simulink library "planarWaveModel_ul"  (R2018b)
settings: Solver=VariableStepAuto  StartTime=0.0  StopTime=10.0  RelTol=1e-3
undefined symbols (not defined in the file): env
settings Model: Creator=jcreed2  LastModifiedBy=jcreed2

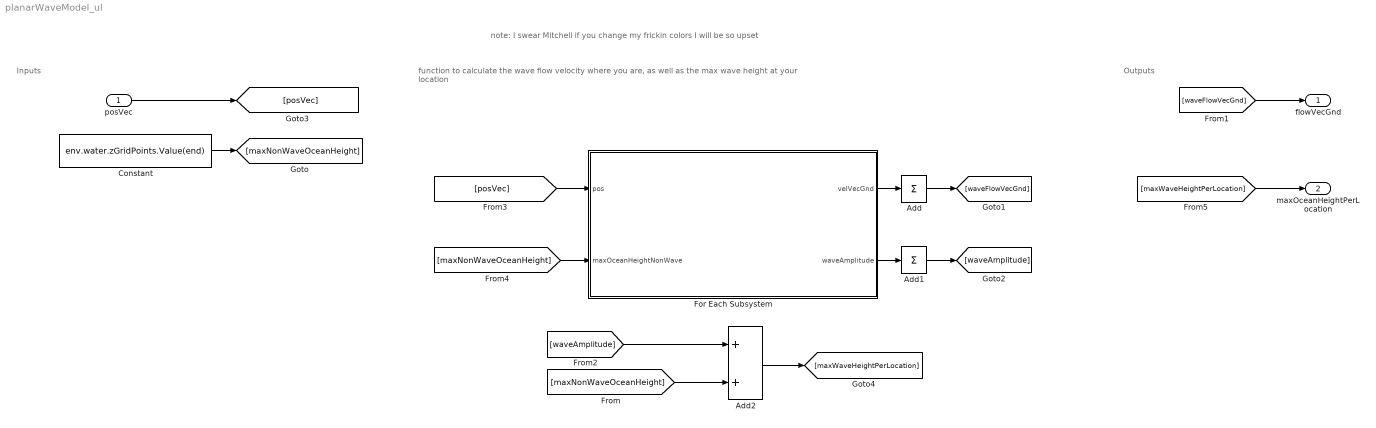
== system planarWaveModel_ul ==
  note: note: I swear Mitchell if you change my frickin colors I will be so upset
  note: Outputs
  note: Inputs
  note: function to calculate the wave flow velocity where you are, as well as the max wave height at your location
  posVec : Inport
  Add : Sum  Inputs=+
  Add1 : Sum  Inputs=+
  Add2 : Sum
  Constant : Constant  Value=env.water.zGridPoints.Value(end)
  For Each Subsystem : Subsystem  TreatAsAtomicUnit=on  mask{waveStruct=env.waterWave.struct('ENV.planarWaveModel')}
      mask prompts: waveStruct "wave structure"
      mask DialogControl Control2 Prompt: Insert wave structure
  "flowVecGnd " : Outport
  maxOceanHeightPerLocation : Outport  Port=2
  wires:
  Constant/1 -> [maxNonWaveOceanHeight]
  For Each Subsystem/1("velVecGnd ") -> Add/1
  For Each Subsystem/2(waveAmplitude) -> Add1/1
  Add/1 -> [waveFlowVecGnd]
  [waveFlowVecGnd] -> "flowVecGnd "/1
  Add1/1 -> [waveAmplitude]
  posVec/1 -> [posVec]
  [posVec] -> For Each Subsystem/1("pos ")
  [waveAmplitude] -> Add2/1
  [maxNonWaveOceanHeight] -> Add2/2
  [maxNonWaveOceanHeight] -> For Each Subsystem/2("maxOceanHeightNonWave ")
  Add2/1 -> [maxWaveHeightPerLocation]
  [maxWaveHeightPerLocation] -> maxOceanHeightPerLocation/1

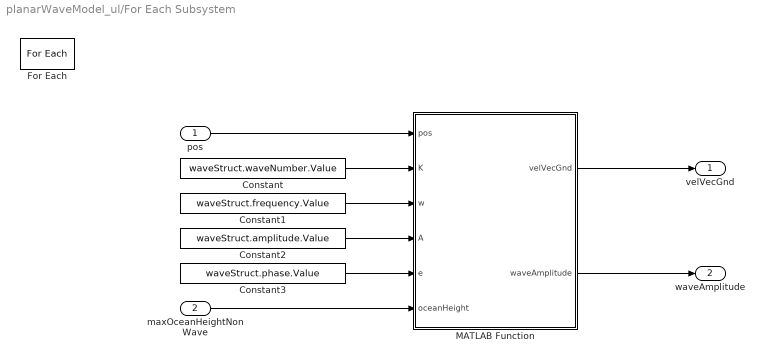
== system planarWaveModel_ul/For Each Subsystem ==
  "pos " : Inport
  "maxOceanHeightNonWave " : Inport  Port=2
  Constant : Constant  Value=waveStruct.waveNumber.Value
  Constant1 : Constant  Value=waveStruct.frequency.Value
  Constant2 : Constant  Value=waveStruct.amplitude.Value
  Constant3 : Constant  Value=waveStruct.phase.Value
  For Each : ForEach  DisableCoverage=on  IterateSubsysMaskParameter=on  SubsysMaskParameterIterationDimension=2  IndexMode=One-based
  MATLAB Function : MATLAB Function  TreatAsAtomicUnit=on
  "velVecGnd " : Outport  ConcatenationDimension=1
  waveAmplitude : Outport  Port=2  ConcatenationDimension=1
  wires:
  MATLAB Function/1(velVecGnd) -> "velVecGnd "/1
  "pos "/1 -> MATLAB Function/1(pos)
  Constant/1 -> MATLAB Function/2(K)
  Constant1/1 -> MATLAB Function/3(w)
  Constant2/1 -> MATLAB Function/4(A)
  Constant3/1 -> MATLAB Function/5(e)
  MATLAB Function/2(waveAmplitude) -> waveAmplitude/1
  "maxOceanHeightNonWave "/1 -> MATLAB Function/6(oceanHeight)

== matlab function planarWaveModel_ul/For Each Subsystem/MATLAB Function ==
  data: pos input; velVecGnd output; K input; w input; A input; e input; waveAmplitude output; oceanHeight input
function [velVecGnd,waveAmplitude] = fcn(pos, K, w, A, e, oceanHeight)

y = u;
